simulink library "ctrlSurfCalc_cl"  (R2020a)
settings: Solver=VariableStepAuto  StartTime=0.0  StopTime=10.0  RelTol=1e-3
undefined symbols (not defined in the file or in its folder): vhcl
libraries: dspstat3 x2, dsppolyfun x2
settings Model: Creator=jcreed2  LastModifiedBy=adabney

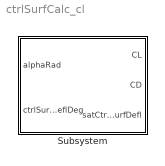
== system ctrlSurfCalc_cl ==
  Subsystem : Subsystem  mask{aSurf=0}
      mask prompts: aSurf "aeroSurf object"

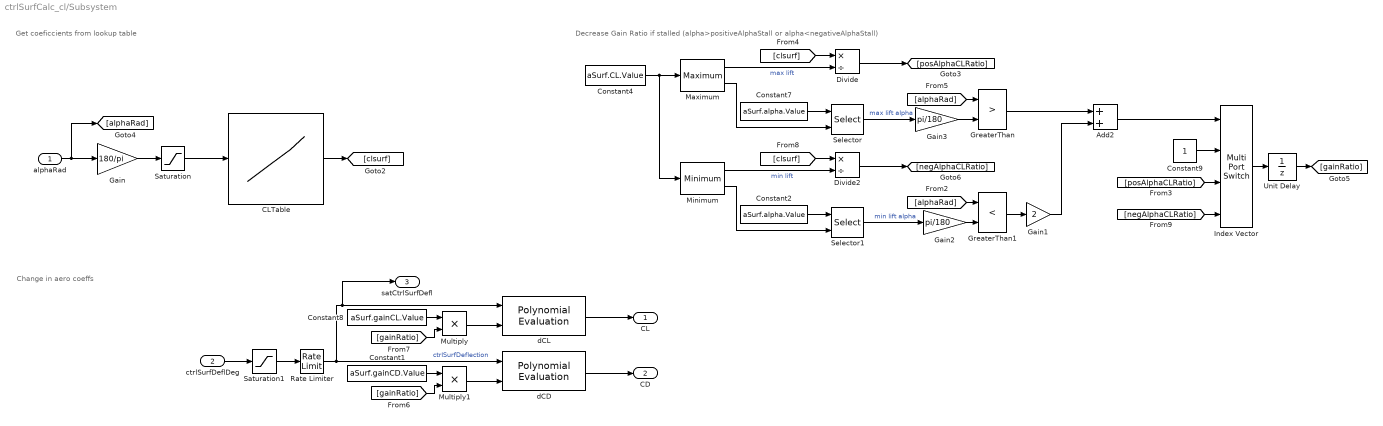
== system ctrlSurfCalc_cl/Subsystem ==
  note: Get coeficcients from lookup table
  note: Change in aero coeffs
  note: Decrease Gain Ratio if stalled (alpha>positiveAlphaStall or alpha<negativeAlphaStall)
  alphaRad : Inport
  ctrlSurfDeflDeg : Inport  Port=2
  Add2 : Sum
  CLTable : Lookup_n-D  NumberOfTableDimensions=1  LookupTableObject=CLTable  BreakpointsForDimension1=aSurf.alpha.Value  Table=aSurf.CL.Value  ExtrapMethod=Clip  UseLastTableValue=on  InternalRulePriority=Speed  RndMeth=Simplest  InputSameDT=on
  Constant1 : Constant  Value=aSurf.gainCD.Value
  Constant2 : Constant  Value=aSurf.alpha.Value
  Constant4 : Constant  Value=aSurf.CL.Value
  Constant7 : Constant  Value=aSurf.alpha.Value
  Constant8 : Constant  Value=aSurf.gainCL.Value
  Constant9 : Constant
  Divide : Product  Inputs=*/
  Divide2 : Product  Inputs=*/
  Gain : Gain  Gain=180/pi
  Gain1 : Gain  Gain=2
  Gain2 : Gain  Gain=pi/180
  Gain3 : Gain  Gain=pi/180
  GreaterThan : RelationalOperator  Operator=>  OutDataTypeStr=boolean  RndMeth=Simplest
  GreaterThan1 : RelationalOperator  Operator=<  OutDataTypeStr=boolean  RndMeth=Simplest
  Index Vector : MultiPortSwitch  DataPortOrder=Zero-based contiguous  zeroidx=on
  Maximum : dspstat3/Maximum  operation=maximum  fcn=Value and Index  indexBase=One  operateOver=Each column  Dimension=1  InputProcessing=Columns as channels (frame based)  reset=None  roiEnable=off  roiType=Rectangles  roiPortion=Entire ROI  roiOutput=Individual statistics for each ROI  roiFlag=off  roundingMode=Floor  overflowMode=off  accumDataTypeStr=Inherit: Same as product output  accumLastDataTypeStr=Inherit: Same as product output
  Minimum : dspstat3/Minimum  operation=minimum  fcn=Value and Index  indexBase=One  operateOver=Each column  Dimension=1  InputProcessing=Columns as channels (frame based)  reset=None  roiEnable=off  roiType=Rectangles  roiPortion=Entire ROI  roiOutput=Individual statistics for each ROI  roiFlag=off  roundingMode=Floor  overflowMode=off
      settings: SourceProductBaseCode=DS
  Multiply : Product
  Multiply1 : Product
  Rate Limiter : RateLimiter  RisingSlewLimit=aSurf.maxCtrlDefSpeed.Value  FallingSlewLimit=-aSurf.maxCtrlDefSpeed.Value  SampleTimeMode=inherited
  Saturation : Saturate  UpperLimit=90  LowerLimit=-90
  Saturation1 : Saturate  UpperLimit=aSurf.maxCtrlDef.Value  LowerLimit=aSurf.minCtrlDef.Value
  Selector : Selector  InputPortWidth=length(vhcl.portWing.alpha.Value)  IndexOptions=Index vector (port)  Indices=[1 3]  OutputSizes=1
  Selector1 : Selector  InputPortWidth=length(vhcl.portWing.alpha.Value)  IndexOptions=Index vector (port)  Indices=[1 3]  OutputSizes=1
  Unit Delay : UnitDelay  InitialCondition=1  SampleTime=-1  HasFrameUpgradeWarning=on
  dCD : dsppolyfun/Polynomial Evaluation  useConstCoeffs=off  constCoeffs=[0]
      settings: SourceProductBaseCode=DS
  dCL : dsppolyfun/Polynomial Evaluation  useConstCoeffs=off  constCoeffs=[0]
      settings: SourceProductBaseCode=DS
  CL : Outport  VectorParamsAs1DForOutWhenUnconnected=off
  CD : Outport  Port=2  VectorParamsAs1DForOutWhenUnconnected=off
  satCtrlSurfDefl : Outport  Port=3
  wires:
  Add2/1 -> Index Vector/1
  Constant1/1 -> Multiply1/1
  Gain2/1 -> GreaterThan1/2
  Maximum/2 -> Selector/2
  Multiply/1 -> dCL/2
  Constant9/1 -> Index Vector/2
  [gainRatio] -> Multiply/2
  [posAlphaCLRatio] -> Index Vector/3
  [alphaRad] -> GreaterThan1/1
  [clsurf] -> Divide/1
  Maximum/1 -> Divide/2  "max lift"
  Selector1/1 -> Gain2/1  "min lift alpha"
  Divide2/1 -> [negAlphaCLRatio]
  Divide/1 -> [posAlphaCLRatio]
  Selector/1 -> Gain3/1  "max lift alpha"
  dCL/1 -> CL/1
  [clsurf] -> Divide2/1
  Constant4/1 -> Minimum/1, Maximum/1
  dCD/1 -> CD/1
  Minimum/2 -> Selector1/2
  GreaterThan1/1 -> Gain1/1
  Rate Limiter/1 -> dCD/1, satCtrlSurfDefl/1, dCL/1  "ctrlSurfDeflection"
  Saturation/1 -> CLTable/1
  Constant2/1 -> Selector1/1
  Minimum/1 -> Divide2/2  "min lift"
  alphaRad/1 -> Gain/1, [alphaRad]
  Constant8/1 -> Multiply/1
  [negAlphaCLRatio] -> Index Vector/4
  Gain/1 -> Saturation/1
  Gain3/1 -> GreaterThan/2
  ctrlSurfDeflDeg/1 -> Saturation1/1
  GreaterThan/1 -> Add2/1
  [alphaRad] -> GreaterThan/1
  Gain1/1 -> Add2/2
  CLTable/1 -> [clsurf]
  Constant7/1 -> Selector/1
  Index Vector/1 -> Unit Delay/1
  [gainRatio] -> Multiply1/2
  Saturation1/1 -> Rate Limiter/1
  Multiply1/1 -> dCD/2
  Unit Delay/1 -> [gainRatio]
